simulink model "signalgeneration"  (Simulink 7.6)
settings: Solver=ode45  StartTime=0.0  StopTime=10.0  RelTol=1e-3
libraries: simulink x3
settings Model: Creator=root  LastModifiedBy=root
settings SolverCC: ShapePreserveControl=EnableAll

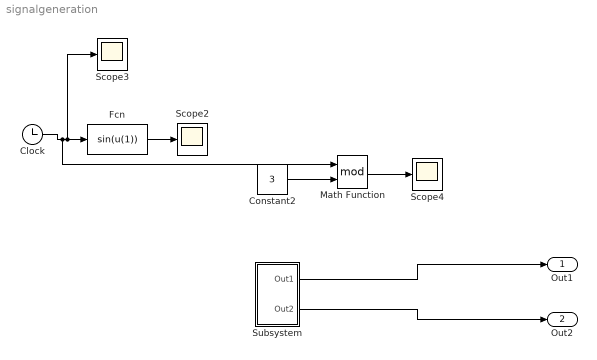
== system signalgeneration ==
  Clock : Clock
      settings: Decimation=10
  Constant2 : Constant  Value=3
  Fcn : Fcn  Expr=sin(u(1))
  Math Function : Math  Operator=mod  SaturateOnIntegerOverflow=on
  Scope2 : Scope
  Scope3 : Scope
      settings: SaveName=ScopeData2
  Scope4 : Scope
      settings: SaveName=ScopeData3
  Subsystem : Subsystem
  Out1 : Outport
  Out2 : Outport  Port=2
  wires:
  Clock/1 -> Fcn/1, Scope3/1, Math Function/1
  Fcn/1 -> Scope2/1
  Constant2/1 -> Math Function/2
  Math Function/1 -> Scope4/1
  Subsystem/1(Out1) -> Out1/1
  Subsystem/2(Out2) -> Out2/1

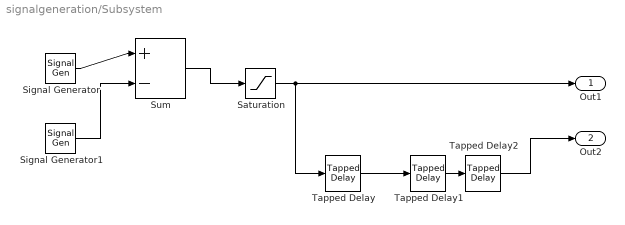
== system signalgeneration/Subsystem ==
  Saturation : Saturate  UpperLimit=1  LowerLimit=0
  Signal Generator : SignalGenerator  WaveForm=square
  Signal Generator1 : SignalGenerator  WaveForm=square  Frequency=0.5
  Sum : Sum  Inputs=|+-
  Tapped Delay : simulink/Discrete/Tapped Delay  vinit=0.0  samptime=-1  NumDelays=1  DelayOrder=Oldest  includeCurrent=off
  Tapped Delay1 : simulink/Discrete/Tapped Delay  vinit=0.0  samptime=-1  NumDelays=1  DelayOrder=Oldest  includeCurrent=off
  Tapped Delay2 : simulink/Discrete/Tapped Delay  vinit=0.0  samptime=-1  NumDelays=1  DelayOrder=Oldest  includeCurrent=off
  Out1 : Outport
  Out2 : Outport  Port=2
  wires:
  Signal Generator/1 -> Sum/1
  Signal Generator1/1 -> Sum/2
  Sum/1 -> Saturation/1
  Saturation/1 -> Tapped Delay/1, Out1/1
  Tapped Delay1/1 -> Tapped Delay2/1
  Tapped Delay/1 -> Tapped Delay1/1
  Tapped Delay2/1 -> Out2/1
